simulink model "W04_P0_second_order"  (R2024b)
settings: Solver=ode4  StartTime=0.0  StopTime=15  FixedStep=0.001  RelTol=1e-3
values from neighbouring files (symbols this model uses):
  wn = sqrt(Kp/Iz)    [W04_pole_place.m]    (also in W04_setup.m = 1.4142)
  zeta = (Nr + Kd) / (2*sqrt(Kp*Iz))    [W04_pole_place.m]    (also in W04_setup.m = 0.7071)
settings Model: Creator=admin  LastModifiedBy=admin

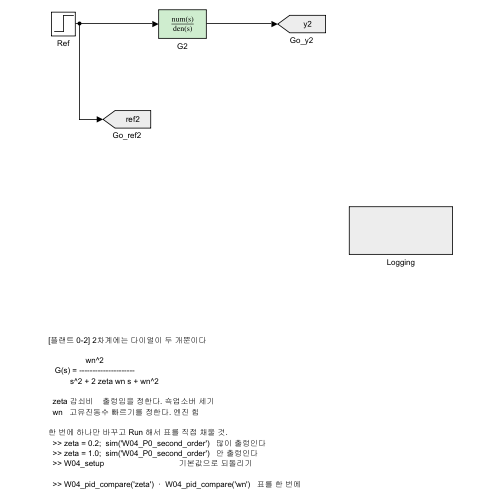
[thumbnail: Simulink's stored preview of the top-level diagram]
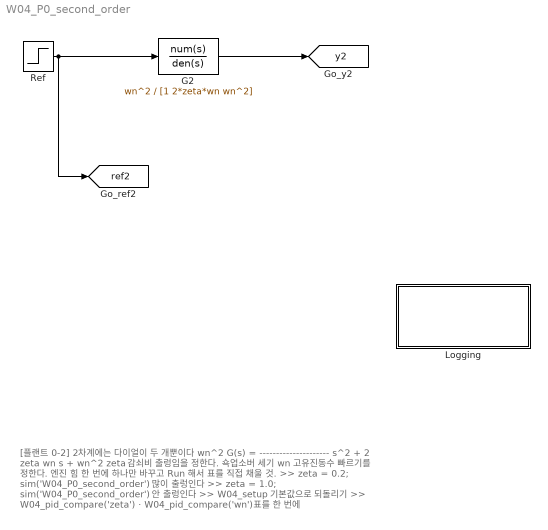
== system W04_P0_second_order ==
  note: [플랜트 0-2] 2차계에는 다이얼이 두 개뿐이다
      |
      |                  wn^2
      |    G(s) = ---------------------
      |           s^2 + 2 zeta wn s + wn^2
      |
      |   zeta 감쇠비    출렁임을 정한다. 쇽업소버 세기
      |   wn   고유진동수 빠르기를 정한다. 엔진 힘
      |
      | 한 번에 하나만 바꾸고 Run 해서 표를 직접 채울 것.
      |   >> zeta = 0.2;  sim('W04_P0_second_order')   많이 출렁인다
      |   >> zeta = 1.0;  sim('W04_P0_second_order')   안 출렁인다
      |   >> W04_setup                                  기본값으로 되돌리기
      |
      |   >> W04_pid_compare('zeta')  ·  W04_pid_compare('wn')   표를 한 번에
  G2 : TransferFcn  Numerator=wn^2  Denominator=[1 2*zeta*wn wn^2]
  Logging : Subsystem
  Ref : Step  SampleTime=0
  tag scope: ref2=global, y2=global
  wires:
  Ref/1 -> G2/1, [ref2]
  G2/1 -> [y2]

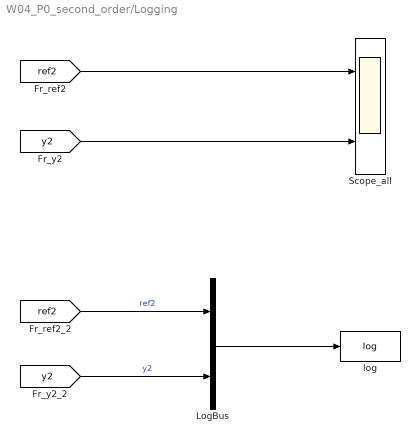
== system W04_P0_second_order/Logging ==
  LogBus : BusCreator  Inputs=2
  Scope_all : Scope  NumInputPorts=2
  log : ToWorkspace  VariableName=log  SaveFormat=Timeseries  SampleTime=-1
  wires:
  [ref2] -> Scope_all/1
  [y2] -> Scope_all/2
  [ref2] -> LogBus/1  "ref2"
  [y2] -> LogBus/2  "y2"
  LogBus/1 -> log/1
